simulink model "gomx3_control"  (R2023a)
settings: Solver=VariableStepAuto  StartTime=0.0  StopTime=1000  RelTol=1e-3  EnableMultiTasking=on
model workspace: external: MAT-File (data not in the file)
libraries: aausat3_lib x7, vrlib x1
settings Model: Creator=jn  LastModifiedBy=jacobel-omar
settings SolverCC: AlgebraicLoopSolver=TrustRegion
settings DataIOCC: SaveFormat=Array  ReturnWorkspaceOutputs=off
settings OptimizationCC: LifeSpan=inf
settings DebuggingCC: SolverPrmCheckMsg=warning  UnconnectedInputMsg=warning  UnconnectedOutputMsg=warning  UnconnectedLineMsg=warning  AllowSymbolicDim=off  SFUnexpectedBacktrackingDiag=warning  SFNoUnconditionalDefaultTransitionDiag=warning  SFExecutionAtInitializationDiag=none  ArithmeticOperatorsInVariantConditions=warning
settings ModelReferenceCC: EnableRefExpFcnMdlSchedulingChecks=on  PropagateSignalLabelsOutOfModel=off
settings SFSimCC: SimUseLocalCustomCode=off  CustomCodeUndefinedFunction=UseInterfaceOnly
settings RTWCC: RTWUseLocalCustomCode=off
settings CodeAppCC: StateflowObjectComments=on
settings GRTTargetCC: TargetLangStandard=C89/C90 (ANSI)
settings ConfigComp: CovMetricSettings=dw  CovSaveCumulativeToWorkspaceVar=on  CovSaveSingleToWorkspaceVar=on  CovExternalEMLEnable=off  CovSFcnEnable=off

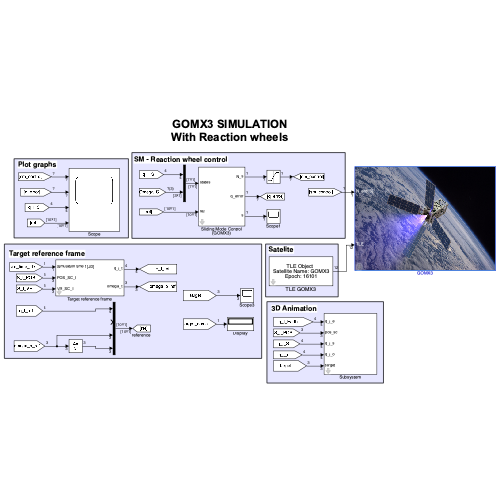
[thumbnail: Simulink's stored preview of the top-level diagram]
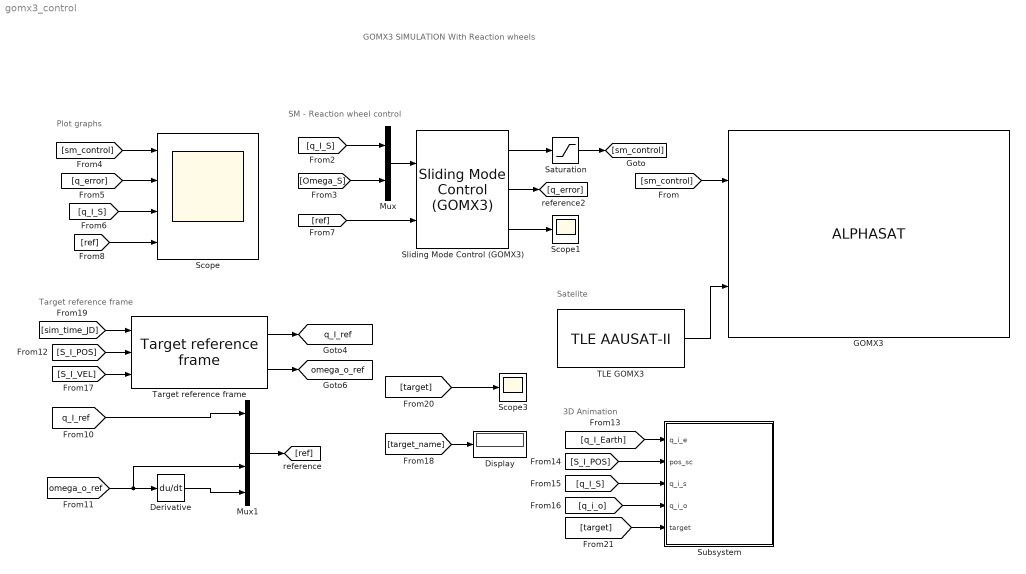
== system gomx3_control ==
  note: GOMX3 SIMULATION
      | With Reaction wheels
  note: Target reference frame
  note: SM - Reaction wheel control
  note: Satelite
  note: 3D Animation
  note: Plot graphs
  Derivative : Derivative
  Display : Display
  GOMX3 : aausat3_lib/ALPHASAT  date='2016-04-10T15:37Z'  q_init_I_S=[0.5 0.5 0.5 0.5]  w_init_S=[0.002,0.002,0.002]  enable_env_disturbance=on  Dim=[0.1 0.1 0.133*3]  sc_mass=0.8*3  r_com=[0 0 0]  inertia_C=[0.0371 0.0371 0.0059]  q_S_C=[0 0 0 1]  Cd=2  rho=5e-14  solar_m_flux=4.5565e-6  solar_absorb_coeff=1.5  mag_dipole=0.001
      settings: SourceProductName=AAUSAT3
  Mux : Mux  Inputs=2
  Mux1 : Mux
  Saturation : Saturate  UpperLimit=23e-6  LowerLimit=-23e-6
  Scope : Scope  NumInputPorts=4
  Scope1 : Scope
  Scope3 : Scope
  Sliding Mode Control (GOMX3) : aausat3_lib/ACS/Sliding Mode Control (GOMX3)  K=diag([1 1 1])*4  delta_0=0.05  e=100e-2  max_disturbance=6.0306e-08  q_s_c=[0 0 0 1]'  Js=[0.0371 0.0371 0.0059]  Ts=1  coriolis_on=on  Jrw=[5.1431e-7 5.1431e-7 7e-7]  q_s_tetra=[0 0 1 0]'
      settings: SourceProductName=AAUSAT3
  Subsystem : Subsystem  mask{Re=6371e3, scale=1000}
      mask prompts: Re "Earth Radius"; scale "Animation scale"
  TLE GOMX3 : aausat3_lib/Orbit and Ephemeris/TLE AAUSAT-II  satname='GOMX3'  JulianDay=16101.77114494  xndt2o=0.00040383  xndd6o=0  bstar=0.30799e-3  xincl=51.6376  xnodeo=21.5314  eo=0.0003860  omegao=1.6250  xmo=358.4760  xno=15.71795136  ts=1
      settings: SourceProductName=AAUSAT3
  Target reference frame : aausat3_lib/Orbit and Ephemeris/Target reference frame  min_elevation=0  Ts=10  target_list='target_list.mat'  enabel_target=on
      settings: SourceProductName=AAUSAT3
  tag scope: omega_o_ref=global, q_I_ref=global
  wires:
  [sm_control] -> Scope/1
  [q_I_ref] -> Mux1/1
  Derivative/1 -> Mux1/4
  [q_error] -> Scope/2
  [q_I_S] -> Scope/3
  Mux1/1 -> [ref]
  [ref] -> Scope/4
  TLE GOMX3/1 -> GOMX3/2
  [omega_o_ref] -> Derivative/1, Mux1/3
  [S_I_VEL] -> Target reference frame/3
  [S_I_POS] -> Target reference frame/2
  [sim_time_JD] -> Target reference frame/1
  [target_name] -> Display/1
  [target] -> Scope3/1
  [q_I_Earth] -> Subsystem/1(q_i_e)
  [S_I_POS] -> Subsystem/2(pos_sc)
  [q_I_S] -> Subsystem/3(q_i_s)
  [q_i_o] -> Subsystem/4(q_i_o)
  [target] -> Subsystem/5(target)
  [sm_control] -> GOMX3/1
  [Omega_S] -> Mux/2
  Mux/1 -> Sliding Mode Control (GOMX3)/1
  [ref] -> Sliding Mode Control (GOMX3)/2
  Sliding Mode Control (GOMX3)/3 -> Scope1/1
  Sliding Mode Control (GOMX3)/2 -> [q_error]
  Sliding Mode Control (GOMX3)/1 -> Saturation/1
  Saturation/1 -> [sm_control]
  [q_I_S] -> Mux/1
  Target reference frame/1 -> [q_I_ref]
  Target reference frame/2 -> [omega_o_ref]

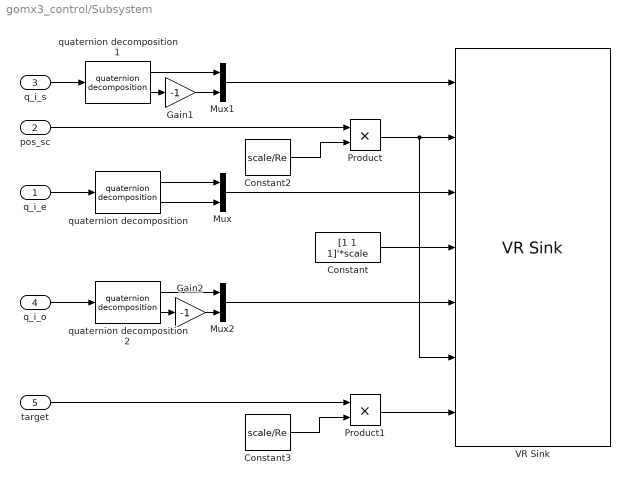
== system gomx3_control/Subsystem ==
  q_i_e : Inport
  pos_sc : Inport  Port=2
  q_i_s : Inport  Port=3
  q_i_o : Inport  Port=4
  target : Inport  Port=5
  Constant : Constant  Value=[1 1 1]'*scale
  Constant2 : Constant  Value=scale/Re
  Constant3 : Constant  Value=scale/Re
  Gain1 : Gain  Gain=-1
  Gain2 : Gain  Gain=-1
  Mux : Mux  Inputs=2
  Mux1 : Mux  Inputs=2
  Mux2 : Mux  Inputs=2
  Product : Product
  Product1 : Product
  VR Sink : vrlib/VR Sink  InstantiateOnLoad=on  SampleTime=0.1  ViewEnable=on  RemoteChange=off  RemoteView=on  FieldsWritten=CubeSat.rotation.4.1.1.double#CubeSat.translation.3.1.1.double#Earth.rotation.4.1.1.double#trans.scale.3.1.1.double#sat_view.rotation.4.1.1.double#sat_view.translation.3.1.1.double#target.translation.3.1.1.double  WorldFileName=lib/utils/animation/sat_orbit.wrl  WorldDescription=The Earth - Low Resolution Model  AutoView=off  VideoDimensions=[]  AllowVariableSize=off
  quaternion decomposition : aausat3_lib/Math Utilities/Quaternion operations/quaternion decomposition  SystemSampleTime=-1  VariantActivationTime=update diagram  Latency=0  AutoFrameSizeCalculation=off
      settings: SourceProductName=AAUSAT3
  quaternion decomposition1 : aausat3_lib/Math Utilities/Quaternion operations/quaternion decomposition  SystemSampleTime=-1  VariantActivationTime=update diagram  Latency=0  AutoFrameSizeCalculation=off
      settings: SourceProductName=AAUSAT3
  quaternion decomposition2 : aausat3_lib/Math Utilities/Quaternion operations/quaternion decomposition  SystemSampleTime=-1  VariantActivationTime=update diagram  Latency=0  AutoFrameSizeCalculation=off
      settings: SourceProductName=AAUSAT3
  wires:
  q_i_e/1 -> quaternion decomposition/1
  quaternion decomposition/2 -> Mux/2
  quaternion decomposition/1 -> Mux/1
  q_i_s/1 -> quaternion decomposition1/1
  quaternion decomposition1/2 -> Gain1/1
  quaternion decomposition1/1 -> Mux1/1
  q_i_o/1 -> quaternion decomposition2/1
  quaternion decomposition2/1 -> Mux2/1
  Gain1/1 -> Mux1/2
  quaternion decomposition2/2 -> Gain2/1
  Gain2/1 -> Mux2/2
  Mux1/1 -> VR Sink/1
  Constant/1 -> VR Sink/4
  pos_sc/1 -> Product/1
  Product/1 -> VR Sink/6, VR Sink/2
  Constant2/1 -> Product/2
  Product1/1 -> VR Sink/7
  Constant3/1 -> Product1/2
  Mux2/1 -> VR Sink/5
  Mux/1 -> VR Sink/3
  target/1 -> Product1/1
